simulink model "model_compare"  (R2023b)
settings: Solver=ode1  StartTime=0.0  StopTime=500  FixedStep=0.002  RelTol=1e-3  EnableMultiTasking=on
libraries: simulink x1
settings Model: Creator=danie  LastModifiedBy=danie
settings SolverCC: AutoInsertRateTranBlk=on  InsertRTBMode=Always

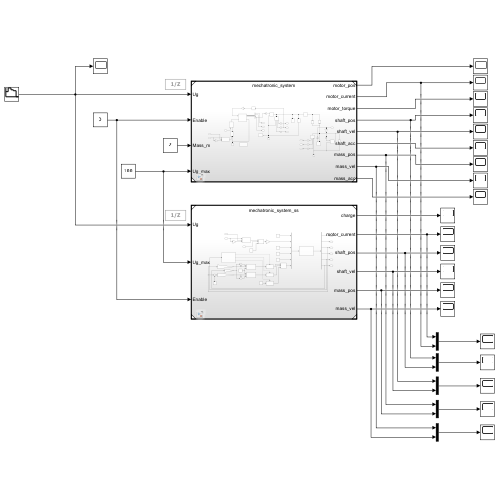
[thumbnail: Simulink's stored preview of the top-level diagram]
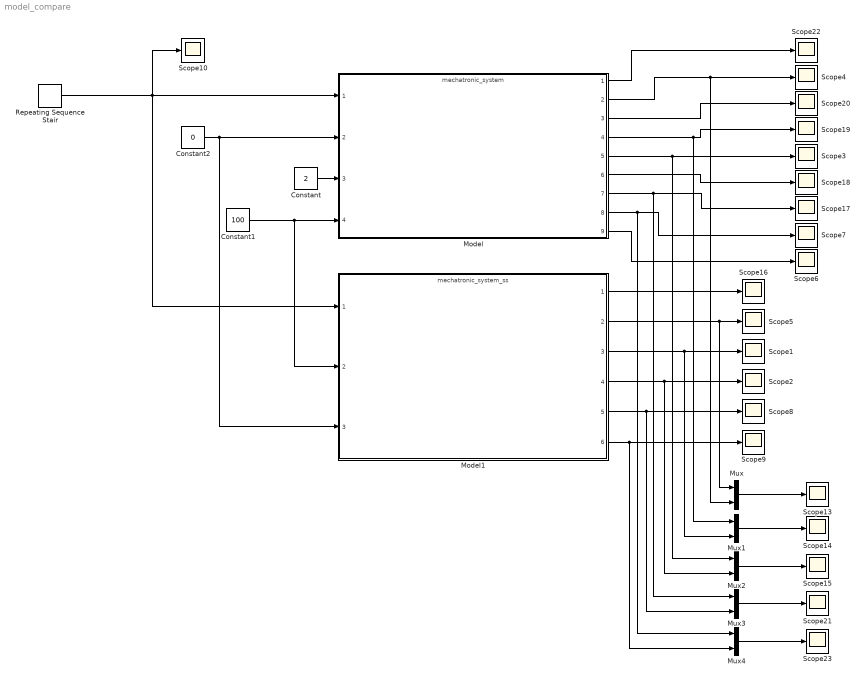
== system model_compare ==
  Constant : Constant  Value=2
  Constant1 : Constant  Value=100
  Constant2 : Constant  Value=0
  Model : ModelReference  ModelNameDialog=mechatronic_system.slx  SimulationMode=Normal  ModelReferenceVersion=1.20
  Model1 : ModelReference  ModelNameDialog=mechatronic_system_ss.slx  SimulationMode=Normal  ModelReferenceVersion=1.12
  Mux{,1..4} (5 alike) : Mux  Inputs=2
  Repeating Sequence Stair : simulink/Sources/Repeating Sequence Stair  OutValues=[10 18 14 12 0].'  tsamp=5  OutMin=[]  OutMax=[]  OutDataTypeStr=double  OutputDataTypeScalingMode=double  OutDataType=fixdt(0,8)  ConRadixGroup=Best Precision: Vector-wise  OutScaling=2^-12
  Scope{1..10,13..23} (21 alike) : Scope
  wires:
  Constant/1 -> Model/3
  Constant1/1 -> Model1/2, Model/4
  Constant2/1 -> Model1/3, Model/2
  Repeating Sequence Stair/1 -> Scope10/1, Model1/1, Model/1
  Model1/3 -> Mux1/2, Scope1/1
  Model1/4 -> Mux2/2, Scope2/1
  Model/5 -> Mux2/1, Scope3/1
  Model1/2 -> Mux/1, Scope5/1
  Model/8 -> Mux4/1, Scope7/1
  Model1/5 -> Mux3/2, Scope8/1
  Model1/6 -> Mux4/2, Scope9/1
  Mux/1 -> Scope13/1
  Mux1/1 -> Scope14/1
  Mux2/1 -> Scope15/1
  Model1/1 -> Scope16/1
  Model/9 -> Scope6/1
  Model/6 -> Scope18/1
  Model/7 -> Mux3/1, Scope17/1
  Model/4 -> Mux1/1, Scope19/1
  Model/3 -> Scope20/1
  Model/2 -> Mux/2, Scope4/1
  Model/1 -> Scope22/1
  Mux4/1 -> Scope23/1
  Mux3/1 -> Scope21/1
